simulink model "OmegaTest"  (R2016a)
settings: Solver=FixedStepAuto  StartTime=0.0  StopTime=inf  FixedStep=0.01  RelTol=1e-11
libraries: xpcseriallib x1, dspnetwork x1
Description:
  | Bringing in C++ Code into a C++ S-function Including Code Generation Support
settings Model: ExtModeTrigMode=oneshot  ExtModeArmWhenConnect=off  ExtModeAutoUpdateStatusClock=off  Creator=The MathWorks Inc.  LastModifiedBy=robotic
settings SolverCC: ZeroCrossControl=EnableAll
settings DataIOCC: SaveFormat=Array  SaveOutput=off  SignalLogging=off  SaveTime=off  SignalLoggingName=logsOut
settings OptimizationCC: ExpressionDepthLimit=2147483647  StateBitsets=on  DataBitsets=on  InitFltsAndDblsToZero=on  BufferReusableBoundary=off
settings DebuggingCC: SaveWithParameterizedLinksMsg=none  UnderspecifiedInitializationDetection=Classic  MergeDetectMultiDrivingBlocksExec=none  SignalResolutionControl=TryResolveAllWithWarning  MultiTaskDSMMsg=warning  MultiTaskCondExecSysMsg=none  SigSpecEnsureSampleTimeMsg=none  FcnCallInpInsideContextMsg=UseLocalSettings  StateNameClashWarn=warning
settings HardwareCC: ProdBitPerPointer=32  ProdLargestAtomicFloat=None  ProdIntDivRoundTo=Undefined  ProdEndianess=Unspecified  ProdWordSize=32  ProdHWDeviceType=Specified  TargetHWDeviceType=32-bit Generic  ProdEqTarget=off
settings ModelReferenceCC: PropagateSignalLabelsOutOfModel=off
settings RTWCC: Description=Generic Real-Time Target  GenerateReport=on  RTWVerbose=off  CustomSourceCode="#include \"sfun_cppcount_cpp.h\""  CustomInclude=../../../../simulink/src  LaunchReport=on  TargetLang=C++
settings CodeAppCC: ForceParamTrailComments=on
settings GRTTargetCC: TargetFcnLib=ansi_tfl_tmw.mat  CombineOutputUpdateFcns=off  GRTInterface=on
settings ConfigComp: CovModelRefEnable=Off

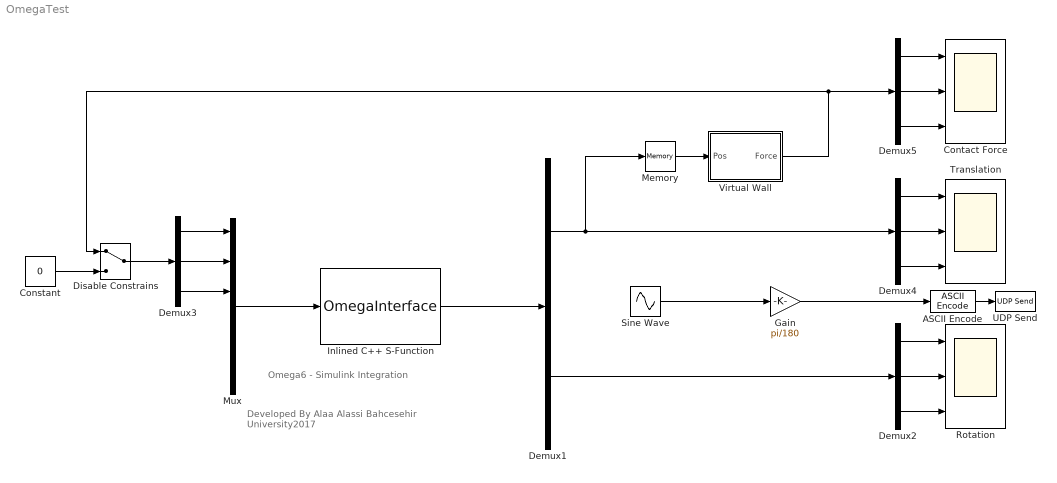
== system OmegaTest ==
  note: Omega6 - Simulink Integration
  note: Developed By Alaa Alassi Bahcesehir University2017
  "ASCII Encode " : xpcseriallib/ASCII Encode   format=%f\n  nvars=1  maxlength=128  vartypes={ 'double' }
  Constant : Constant  Value=0
  Contact Force : Scope  NumInputPorts=3
  Demux1 : Demux  Outputs=2
  Demux{2..5} (4 alike) : Demux  Outputs=3
  Disable Constrains : ManualSwitch
  Gain : Gain  Gain=pi/180
  Inlined C++ S-Function : S-Function  FunctionName=OmegaInterface  SFunctionDeploymentMode=off  EnableBusSupport=off
      mask Display: disp('Inlined C++\nS-Function');
  Memory : Memory
  Mux : Mux  Inputs=6
  Rotation : Scope  NumInputPorts=3
  Sine Wave : Sin  Amplitude=10  Frequency=0.2  SampleTime=0.01
  Translation : Scope  NumInputPorts=3
  UDP Send : dspnetwork/UDP Send  remoteURL='10.2.0.200'  remotePort=2052  localURL='0.0.0.0'  localPortSource=Automatically determine  localPort=-1  sampletime=-1  separateLengthPort=0
  Virtual Wall : MATLAB Function  TreatAsAtomicUnit=on
  wires:
  Demux4/1 -> Translation/1
  Demux4/3 -> Translation/3
  Demux4/2 -> Translation/2
  Demux2/1 -> Rotation/1
  Demux2/3 -> Rotation/3
  Demux2/2 -> Rotation/2
  Demux1/2 -> Demux2/1
  Demux1/1 -> Demux4/1, Memory/1
  Inlined C++ S-Function/1 -> Demux1/1
  Mux/1 -> Inlined C++ S-Function/1
  Constant/1 -> Disable Constrains/2
  Virtual Wall/1(Force) -> Demux5/1, Disable Constrains/1
  Memory/1 -> Virtual Wall/1(Pos)
  Demux3/1 -> Mux/1
  Demux3/2 -> Mux/2
  Demux3/3 -> Mux/3
  Disable Constrains/1 -> Demux3/1
  Demux5/1 -> Contact Force/1
  Demux5/2 -> Contact Force/2
  Demux5/3 -> Contact Force/3
  "ASCII Encode "/1 -> UDP Send/1
  Gain/1 -> "ASCII Encode "/1
  Sine Wave/1 -> Gain/1

== matlab function OmegaTest/Virtual Wall ==
  data: Pos input; Force output
function Force = fcn(Pos)
% Ths function generates a three virtual orthogonal walls that constrains
% the motion of Omega along the three translational drections X,Y and Z.

Borders = [-0.02,-0.02,-0.02]; % in meters
stiffness = 800; % N/m
Force = Constain3D(Pos,Borders,stiffness);

end
